simulink model "doc_rscoding"  (Simulink 6.0)
settings: Solver=ode45  StartTime=0.0  StopTime=500  RelTol=1e-3
undefined symbols (not defined in the file): rsgenpoly, slcm
libraries: commblkcod2 x2, dspbuff3 x2, commrandsrc2 x1
settings Model: Creator=ptrow  LastModifiedBy=agaltman  ProdHWDeviceType=Specified
settings DataIOCC: SignalLoggingName=logsOut
settings OptimizationCC: BlockReduction=off  BooleanDataType=off  MultiInstanced=off
settings FormatCC: IgnoreBidirectionalLines=off
settings HardwareCC: ProdHWDeviceType=Specified
settings CodeAppCC: FileBanners=off  CustomSymbols=off  MangleLength=5
settings GRTTargetCC: TargetFcnLib=iso_c_tmw.mat  IsERTTarget=off

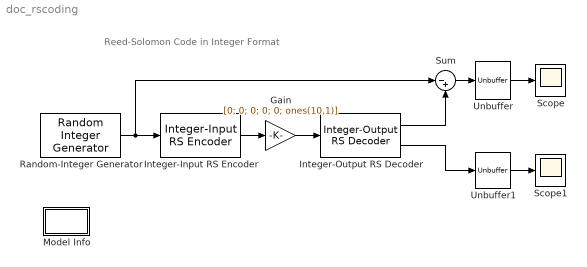
== system doc_rscoding ==
  note: Reed-Solomon Code in Integer Format
  Gain : Gain  Gain=[0; 0; 0; 0; 0; ones(10,1)]  SaturateOnIntegerOverflow=on
  Integer-Input RS Encoder : commblkcod2/Integer-Input RS Encoder  n=15  k=5  specPrimPoly=off  primPoly=[1 0 1 1]  specGenPoly=off  genPoly=rsgenpoly(7,3)
  Integer-Output RS Decoder : commblkcod2/Integer-Output RS Decoder  n=15  k=5  specPrimPoly=off  primPoly=[1 0 1 1]  specGenPoly=off  genPoly=rsgenpoly(7,3)  showNumErr=on
  Model Info : Subsystem  LoadFcn=slcm LoadBlock;  InitFcn=slcm('UpdateAllCMBlocksInThisModelInit')  mask(CMBlock){InitialSaveTempField=, InitialBlockCM=none, BlockCM=none, Frame=on, SaveTempField=, DisplayStringWithTags=Info, MaskDisplayString=Info, HorizontalTextAlignment=Center, LeftAlignmentValue=0.5, SourceBlockDiagram=doc_rscoding, TagMaxNumber=20, CMTag1=, CMTag2=, CMTag3=, CMTag4=, CMTag5=, CMTag6=, CMTag7=, CMTag8=, CMTag9=, CMTag10=, CMTag11=, CMTag12=, CMTag13=, CMTag14=, CMTag15=, CMTag16=, CMTag17=, CMTag18=, CMTag19=, CMTag20=}
      mask help: This block allows revision control information to be displayed within the model.
      settings: CopyFcn=slcm CopyBlock;  DeleteFcn=slcm Cancel;  PostSaveFcn=slcm('UpdateAllCMBlocksInThisModel')  NameChangeFcn=slcm Rename;  OpenFcn=commdemohelp;
      mask Display: text(str2num(LeftAlignmentValue), 0.5, MaskDisplayString, 'HorizontalAlignment', HorizontalTextAlignment)
  Random-Integer Generator : commrandsrc2/Random Integer Generator  mul=15  seed=68521  Ts=1  frameBased=on  sampPerFrame=5  orient=off
  Scope : Scope
  Scope1 : Scope
      settings: YMin=0  YMax=6
  Sum : Sum  Inputs=|-+  SaturateOnIntegerOverflow=on  InputSameDT=on
  Unbuffer : dspbuff3/Unbuffer  ic=0
  Unbuffer1 : dspbuff3/Unbuffer  ic=0
  wires:
  Sum/1 -> Unbuffer/1
  Integer-Input RS Encoder/1 -> Gain/1
  Gain/1 -> Integer-Output RS Decoder/1
  Integer-Output RS Decoder/1 -> Sum/2
  Random-Integer Generator/1 -> Integer-Input RS Encoder/1, Sum/1
  Integer-Output RS Decoder/2 -> Unbuffer1/1
  Unbuffer/1 -> Scope/1
  Unbuffer1/1 -> Scope1/1

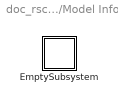
== system doc_rscoding/Model Info ==
  EmptySubsystem : Subsystem

== system doc_rscoding/Model Info/EmptySubsystem ==
